simulink model "balance_simple"  (Simulink 7.0)
settings: Solver=ode45  StartTime=0.0  StopTime=10.0  RelTol=1e-3
values from neighbouring files (symbols this model uses):
  c = 0.08    [bike_linmod.m]    (also in cartpend.m = 0.1; hw2_1a.m = 100; hw3_1b.m = 10; hw3_3a.m = 0.1)
  g = 9.81    [bike_linmod.m]    (also in cartpend.m = 9.8; cruisedyn.m = 9.8; hw2_2.m = 9.8; hw2_2_2.m = 9.8)
  gamma = c*sin(lambda)/b    [bike_linmod.m]    (also in cartpend.m = 0.01; hw3_3a.m = 0.01; hw3_3b.m = 0.01; hw3_3b_2.m = 0.01)
  J = 100    [cartpend.m]    (also in hw3_3a.m; hw3_3b.m; hw3_3b_2.m; hw7_4.m = 0.0475)
  l = 1    [hw3_3a.m]    (also in hw3_3b.m; hw3_3b_2.m; hw7_4.m = 0.05)
  M = [Jxxt -Flx-gamma*Jxzt;-Flx-gamma*Jxzt Fll+2*gamma*Flz+gamma^2*Jzzt]    [bike_linmod.m]    (also in cartpend.m = 10; hw3_3a.m = 10; hw3_3b.m = 10; hw3_3b_2.m = 10)
  m = 80    [cartpend.m]    (also in hw1_3c.m = 1; hw2_1a.m = 1000; hw2_2.m = 1000; hw2_2_2.m = 1000)
undefined symbols (not defined in the file or in its folder): magnitude
settings Model: Creator=george  LastModifiedBy=Douglas MacMynowski  ExtModeAutoUpdateStatusClock=off
settings DataIOCC: SignalLoggingName=sigsOut
settings OptimizationCC: BooleanDataType=off
settings DebuggingCC: SaveWithParameterizedLinksMsg=none  SignalResolutionControl=TryResolveAllWithWarning  SolverPrmCheckMsg=none  MultiTaskDSMMsg=warning  MultiTaskCondExecSysMsg=none  StrictBusMsg=None
settings HardwareCC: TargetUnknown=on
settings RTWCC: IncludeERTFirstTime=on
settings GRTTargetCC: TargetFcnLib=ansi_tfl_tmw.mat

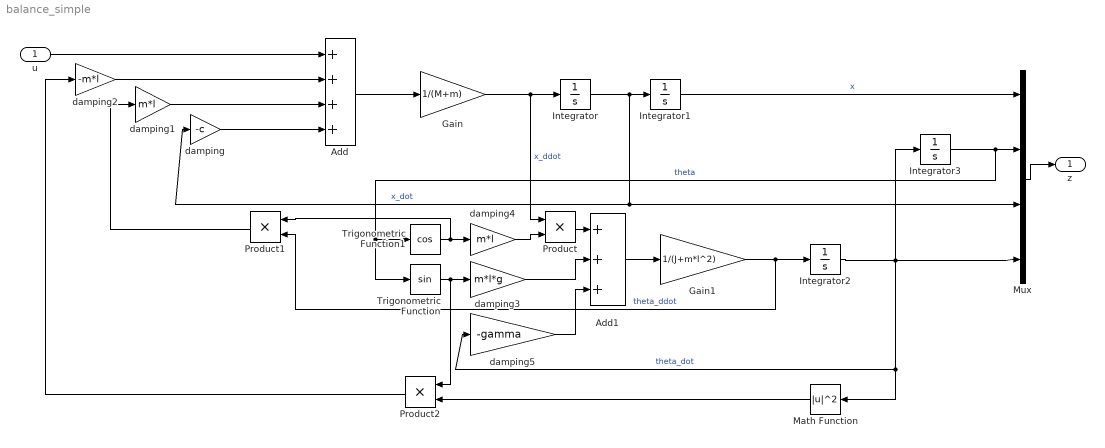
== system balance_simple ==
  u : Inport  OutDataType=sfix(16)  OutScaling=2^0
  Add : Sum  Inputs=++++  OutDataType=sfix(16)  OutScaling=2^-10
  Add1 : Sum  Inputs=+++  OutDataType=sfix(16)  OutScaling=2^-10
  Gain : Gain  Gain=1/(M+m)  ParameterDataType=sfix(16)  ParameterScaling=2^0  OutDataType=sfix(16)  OutScaling=2^0
  Gain1 : Gain  Gain=1/(J+m*l^2)  ParameterDataType=sfix(16)  ParameterScaling=2^0  OutDataType=sfix(16)  OutScaling=2^0
  Integrator{,1..3} (4 alike) : Integrator
  Math Function : Math  Orientation=left  Operator=magnitude^2  OutDataType=sfix(16)  OutScaling=2^0  SaturateOnIntegerOverflow=on
  Mux : Mux
  Product : Product  OutDataType=sfix(16)  OutScaling=2^0  RndMeth=Zero
  Product1 : Product  Orientation=left  OutDataType=sfix(16)  OutScaling=2^0  RndMeth=Zero
  Product2 : Product  Orientation=left  OutDataType=sfix(16)  OutScaling=2^0  RndMeth=Zero
  Trigonometric Function : Trigonometry
  Trigonometric Function1 : Trigonometry  Operator=cos
  damping : Gain  Gain=-c  ParameterDataType=sfix(16)  ParameterScaling=2^0  OutDataType=sfix(16)  OutScaling=2^0
  damping1 : Gain  Gain=m*l  ParameterDataType=sfix(16)  ParameterScaling=2^0  OutDataType=sfix(16)  OutScaling=2^0
  damping2 : Gain  Gain=-m*l  ParameterDataType=sfix(16)  ParameterScaling=2^0  OutDataType=sfix(16)  OutScaling=2^0
  damping3 : Gain  Gain=m*l*g  ParameterDataType=sfix(16)  ParameterScaling=2^0  OutDataType=sfix(16)  OutScaling=2^0
  damping4 : Gain  Gain=m*l  ParameterDataType=sfix(16)  ParameterScaling=2^0  OutDataType=sfix(16)  OutScaling=2^0
  damping5 : Gain  Gain=-gamma  ParameterDataType=sfix(16)  ParameterScaling=2^0  OutDataType=sfix(16)  OutScaling=2^0
  z : Outport  OutDataType=sfix(16)  OutScaling=2^0
  wires:
  Mux/1 -> z/1
  u/1 -> Add/1
  damping1/1 -> Add/3
  Add/1 -> Gain/1
  Gain/1 -> Integrator/1, Product/1  "x_ddot"
  Integrator/1 -> Integrator1/1, Mux/3, damping/1  "x_dot"
  Integrator1/1 -> Mux/1  "x"
  damping/1 -> Add/4
  damping2/1 -> Add/2
  Trigonometric Function/1 -> damping3/1, Product2/1
  Trigonometric Function1/1 -> damping4/1, Product1/1
  Add1/1 -> Gain1/1
  damping3/1 -> Add1/2
  damping4/1 -> Product/2
  Product/1 -> Add1/1
  Gain1/1 -> Integrator2/1, Product1/2  "theta_ddot"
  Integrator2/1 -> Integrator3/1, Mux/4, Math Function/1, damping5/1  "theta_dot"
  Integrator3/1 -> Mux/2, Trigonometric Function/1, Trigonometric Function1/1  "theta"
  Math Function/1 -> Product2/2
  Product2/1 -> damping2/1
  Product1/1 -> damping1/1
  damping5/1 -> Add1/3
